simulink model "Satellite_Attitude_Model"  (R2018b)
settings: Solver=ode23tb  StartTime=0.0  StopTime=1000  FixedStep=0.001  RelTol=1e-4
values from neighbouring files (symbols this model uses):
  A = [A11, A12; A21, A22]    [Satellite_Attitude_Model_Parameters.m]
  ArgOfPerigee_init = deg2rad (TLE_degree(5))    [Satellite_Attitude_Model_Parameters.m]
  b = 10e-6    (= 1e-05)    [Satellite_Attitude_Model_Parameters.m]
  B = [B11,B12; B21,B22]    [Satellite_Attitude_Model_Parameters.m]
  D = 0    [Satellite_Attitude_Model_Parameters.m]
  eccentricity_init = TLE_degree(4)    [Satellite_Attitude_Model_Parameters.m]
  Hconf4 = [Hgyro;Hstr]    [Satellite_Attitude_Model_Parameters.m]
  inclination_init = deg2rad (TLE_degree(2))    [Satellite_Attitude_Model_Parameters.m]
  Km = 0.1    [Satellite_Attitude_Model_Parameters.m]
  Kt = 0.1    [Satellite_Attitude_Model_Parameters.m]
  L = 5.2e-3    (= 0.0052)    [Satellite_Attitude_Model_Parameters.m]
  MeanAnomaly_init = deg2rad (TLE_degree(6))    [Satellite_Attitude_Model_Parameters.m]
  meanMotion_init = meanMotion_init*2*pi/86400    [Satellite_Attitude_Model_Parameters.m]
  Q = 1e-10    [Satellite_Attitude_Model_Parameters.m]
  q_init = [0; 0; 0; 1]    [Satellite_Attitude_Model_Parameters.m]
  R = 2    [Satellite_Attitude_Model_Parameters.m]    (also in dynamicFunctions2.m = 7078000)
  RAAN_init = deg2rad (TLE_degree(3))    [Satellite_Attitude_Model_Parameters.m]
  Rconf4 = [diag(ones(3,1))*Rgyro zeros(3,4);         zeros(4,3) diag(ones(1,4))*Rstr]    [Satellite_Attitude_Model_Parameters.m]
  Rgyro = 1e-12    [Satellite_Attitude_Model_Parameters.m]
  Rstr = 1e-12    [Satellite_Attitude_Model_Parameters.m]
  rw_Inertia = 5e-4    (= 0.0005)    [Satellite_Attitude_Model_Parameters.m]
  RW_Mmax = 0.015    [Satellite_Attitude_Model_Parameters.m]
  rw_SensorToBody = [0 0.4741 0.4741 -0.9482;                   -0.9999 0.3333 0.3333 0.3333;                    0 -0.8165 0.8165 0 ]    [Satellite_Attitude_Model_Parameters.m]
  RW_wmax = 300    [Satellite_Attitude_Model_Parameters.m]
  satInertia = [Isx 0 0 ; 0 Isy 0 ; 0 0 Isz]    [Satellite_Attitude_Model_Parameters.m]    (also in dynamicFunctions2.m = diag([Isx Isy Isz]))
  semimajor_init = sqrt(mu_earth^(1/3)/meanMotion_init^(2/3))    [Satellite_Attitude_Model_Parameters.m]
  Ts = 0.01    [Satellite_Attitude_Model_Parameters.m]
  unit7 = ones(7,1)    [Satellite_Attitude_Model_Parameters.m]
  w_dot_init = [0;0;0]    [Satellite_Attitude_Model_Parameters.m]
  w_init = [0; 0; 0]    [Satellite_Attitude_Model_Parameters.m]
  wRW_init = [0;0;0;0]    [Satellite_Attitude_Model_Parameters.m]
undefined symbols (not defined in the file or in its folder): Continuous, Earth, Time, WGS84
libraries: simulink x14, simulink_extras x13, sharedtransform x8, aerolibutil x2, sharedTrackingLibrary x1, ctrlSharedLib x1, aerolibtransform2 x1, aerolibgravity2 x1
(part 1 of 3)
settings Model: SimulationMode=accelerator  Creator=user  LastModifiedBy=user
settings SolverCC: ZeroCrossControl=DisableAll
settings OptimizationCC: BlockReduction=off  DefaultParameterBehavior=Inlined  BufferReuse=off

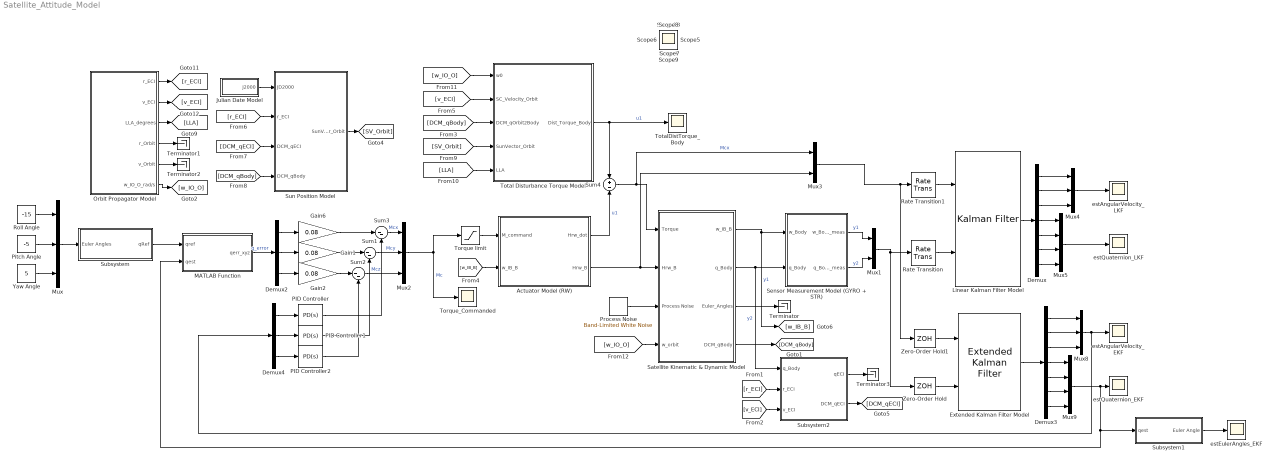
== system Satellite_Attitude_Model ==
  Actuator Model (RW) : Subsystem
  Demux : Demux  Outputs=7
  Demux2 : Demux  Outputs=3
  Demux3 : Demux  Outputs=7
  Demux4 : Demux  Outputs=3
  "Extended Kalman Filter Model " : sharedTrackingLibrary/Extended Kalman Filter  StateTransitionFcn=dynamicFunctions2  HasStateTransitionJacobianFcn=off  HasAdditiveProcessNoise=Additive  ProcessNoise=diag(unit7)*Q  HasTimeVaryingProcessNoise=off  HasStateTransitionFcnExtraArgument=1  InitialState=[w_init; q_init]  InitialStateCovariance=1e-6  MeasurementFcn1=measurementFunction2  HasMeasurementJacobianFcn1=off  HasMeasurementEnablePort1=off  HasAdditiveMeasurementNoise1=Additive  MeasurementNoise1=Rconf4  HasTimeVaryingMeasurementNoise1=off  HasMeasurementFcnExtraArgument1=0  MeasurementFcn2=myMeasurementFcn  HasMeasurementJacobianFcn2=off  HasMeasurementEnablePort2=off  HasAdditiveMeasurementNoise2=Additive  MeasurementNoise2=1  HasTimeVaryingMeasurementNoise2=off  HasMeasurementFcnExtraArgument2=0  MeasurementFcn3=myMeasurementFcn  HasMeasurementJacobianFcn3=off  HasMeasurementEnablePort3=off  HasAdditiveMeasurementNoise3=Additive  MeasurementNoise3=1  HasTimeVaryingMeasurementNoise3=off  HasMeasurementFcnExtraArgument3=0  MeasurementFcn4=myMeasurementFcn  HasMeasurementJacobianFcn4=off  HasMeasurementEnablePort4=off  HasAdditiveMeasurementNoise4=Additive  MeasurementNoise4=1  HasTimeVaryingMeasurementNoise4=off  HasMeasurementFcnExtraArgument4=0  MeasurementFcn5=myMeasurementFcn  HasMeasurementJacobianFcn5=off  HasMeasurementEnablePort5=off  HasAdditiveMeasurementNoise5=Additive  MeasurementNoise5=1  HasTimeVaryingMeasurementNoise5=off  HasMeasurementFcnExtraArgument5=0  EnableMultirate=off  StateTransitionFcnSampleTime=1  MeasurementFcn1SampleTime=1  MeasurementFcn2SampleTime=1  MeasurementFcn3SampleTime=1  MeasurementFcn4SampleTime=1  MeasurementFcn5SampleTime=1  UseCurrentEstimator=on  OutputStateCovariance=off  DataType=double  SampleTime=Ts  NumberOfMeasurements=1
      settings: SourceProductName=Control System Toolbox  SourceProductBaseCode=CT
  Gain1 : Gain  Gain=0.08
  Gain2 : Gain  Gain=0.08
  Gain6 : Gain  Gain=0.08
  Julian Date Model : Subsystem
  Linear Kalman Filter Model : ctrlSharedLib/Kalman Filter  TimeDomain=Continuous-Time  UseCurrentEstimator=on  ModelSource=Individual A, B, C, D matrices  ModelSourceVariable=ss(0.95,1,1,0,1)  A=A  B=B  C=Hconf4  D=D  NumberOfStates=1  NumberOfInputs=1  NumberOfOutputs=1  InitialEstimateSource=Dialog  X0=[w_init; q_init]  P0=10  UseK=off  UseGH=off  NumberOfProcessNoiseInputs=1  G=1  TimeInvariantG=on  H=0  TimeInvariantH=on  Q=diag(unit7)*Q  TimeInvariantQ=on  R=Rconf4  TimeInvariantR=on  N=0  TimeInvariantN=on  AddInputPort=on  AddEnablePort=off  OutputEstimatedY=off  OutputP=off  Ts=-1
      settings: SourceProductBaseCode=CT
  MATLAB Function : MATLAB Function  TreatAsAtomicUnit=on
  Mux{,2,4,8} (4 alike) : Mux  Inputs=3
  Mux1 : Mux  Inputs=2
  Mux3 : Mux  Inputs=2
  Mux5 : Mux
  Mux9 : Mux
  Orbit Propagator Model : Subsystem
  PID Controller : simulink/Continuous/PID Controller  Controller=PD  Form=Parallel  TimeDomain=Continuous-time  SampleTime=-1  IntegratorMethod=Forward Euler  FilterMethod=Forward Euler  ControllerParametersSource=internal  P=1  I=2  D=2  UseFilter=on  N=100  TunerSelectOption=Transfer Function Based (PID Tuner App)  InitialConditionSource=internal  InitialConditionForIntegrator=0  InitialConditionForFilter=0  DifferentiatorICPrevScaledInput=0  ExternalReset=none  TrackingMode=off  Kt=1  LimitOutput=off  UpperSaturationLimit=inf  LowerSaturationLimit=-inf  LinearizeAsGain=on  AntiWindupMode=none  Kb=1  POutMin=[]  POutMax=[]  IOutMin=[]  IOutMax=[]  DOutMin=[]  DOutMax=[]  NOutMin=[]  NOutMax=[]  SumOutMin=[]  SumOutMax=[]  SaturationOutMin=[]  SaturationOutMax=[]  PParamMin=[]  PParamMax=[]  IParamMin=[]  IParamMax=[]  DParamMin=[]  DParamMax=[]  NParamMin=[]  NParamMax=[]  KbParamMin=[]  KbParamMax=[]  KtParamMin=[]  KtParamMax=[]  KbOutMin=[]  KbOutMax=[]  KtOutMin=[]  KtOutMax=[]  IntegratorOutMin=[]  IntegratorOutMax=[]  FilterOutMin=[]  FilterOutMax=[]  SumI1OutMin=[]  SumI1OutMax=[]  SumI2OutMin=[]  SumI2OutMax=[]  SumI3OutMin=[]  SumI3OutMax=[]  SumI4OutMin=[]  SumI4OutMax=[]  SumDOutMin=[]  SumDOutMax=[]  DifferentiatorOutMin=[]  DifferentiatorOutMax=[]  FilterDiffOutCoefMin=[]  FilterDiffOutCoefMax=[]  ReciprocalOutMin=[]  ReciprocalOutMax=[]  SumDenOutMin=[]  SumDenOutMax=[]  SumNumOutMin=[]  SumNumOutMax=[]  DivideOutMin=[]  DivideOutMax=[]  IntegratorContinuousStateAttributes=''  IntegratorStateMustResolveToSignalObject=off  IntegratorRTWStateStorageClass=Auto  FilterContinuousStateAttributes=''  FilterStateMustResolveToSignalObject=off  FilterRTWStateStorageClass=Auto  ParallelPVariant=InternalParameters  IdealPVariant=Disabled  IVariant=Disabled  DVariant=InternalParameters  IntegratorVariant=Disabled  SatVariant=Disabled  AWVariant=Disabled  PCopyVariant=Disabled  TRVariant=Disabled  FdbkBlocksVariant=Forward  IdealPFdbkVariant=Disabled  SatFdbkVariant=Disabled  DerivativeFilterVariant=ContFilter  NVariant=InternalParameters  NCopyVariant=Disabled  FilterICVariant=InternalICsFilter  IntegratorICVariant=Disabled  ExternalResetVariant=Disabled  TRSumVariant=Passthrough  SumFdbkVariant=Disabled  SumVariant=Sum_PD
  PID Controller1 : simulink/Continuous/PID Controller  Controller=PD  Form=Parallel  TimeDomain=Continuous-time  SampleTime=-1  IntegratorMethod=Forward Euler  FilterMethod=Forward Euler  ControllerParametersSource=internal  P=1  I=2  D=2  UseFilter=on  N=100  TunerSelectOption=Transfer Function Based (PID Tuner App)  InitialConditionSource=internal  InitialConditionForIntegrator=0  InitialConditionForFilter=0  DifferentiatorICPrevScaledInput=0  ExternalReset=none  TrackingMode=off  Kt=1  LimitOutput=off  UpperSaturationLimit=inf  LowerSaturationLimit=-inf  LinearizeAsGain=on  AntiWindupMode=none  Kb=1  POutMin=[]  POutMax=[]  IOutMin=[]  IOutMax=[]  DOutMin=[]  DOutMax=[]  NOutMin=[]  NOutMax=[]  SumOutMin=[]  SumOutMax=[]  SaturationOutMin=[]  SaturationOutMax=[]  PParamMin=[]  PParamMax=[]  IParamMin=[]  IParamMax=[]  DParamMin=[]  DParamMax=[]  NParamMin=[]  NParamMax=[]  KbParamMin=[]  KbParamMax=[]  KtParamMin=[]  KtParamMax=[]  KbOutMin=[]  KbOutMax=[]  KtOutMin=[]  KtOutMax=[]  IntegratorOutMin=[]  IntegratorOutMax=[]  FilterOutMin=[]  FilterOutMax=[]  SumI1OutMin=[]  SumI1OutMax=[]  SumI2OutMin=[]  SumI2OutMax=[]  SumI3OutMin=[]  SumI3OutMax=[]  SumI4OutMin=[]  SumI4OutMax=[]  SumDOutMin=[]  SumDOutMax=[]  DifferentiatorOutMin=[]  DifferentiatorOutMax=[]  FilterDiffOutCoefMin=[]  FilterDiffOutCoefMax=[]  ReciprocalOutMin=[]  ReciprocalOutMax=[]  SumDenOutMin=[]  SumDenOutMax=[]  SumNumOutMin=[]  SumNumOutMax=[]  DivideOutMin=[]  DivideOutMax=[]  IntegratorContinuousStateAttributes=''  IntegratorStateMustResolveToSignalObject=off  IntegratorRTWStateStorageClass=Auto  FilterContinuousStateAttributes=''  FilterStateMustResolveToSignalObject=off  FilterRTWStateStorageClass=Auto  ParallelPVariant=InternalParameters  IdealPVariant=Disabled  IVariant=Disabled  DVariant=InternalParameters  IntegratorVariant=Disabled  SatVariant=Disabled  AWVariant=Disabled  PCopyVariant=Disabled  TRVariant=Disabled  FdbkBlocksVariant=Forward  IdealPFdbkVariant=Disabled  SatFdbkVariant=Disabled  DerivativeFilterVariant=ContFilter  NVariant=InternalParameters  NCopyVariant=Disabled  FilterICVariant=InternalICsFilter  IntegratorICVariant=Disabled  ExternalResetVariant=Disabled  TRSumVariant=Passthrough  SumFdbkVariant=Disabled  SumVariant=Sum_PD
  PID Controller2 : simulink/Continuous/PID Controller  Controller=PD  Form=Parallel  TimeDomain=Continuous-time  SampleTime=-1  IntegratorMethod=Forward Euler  FilterMethod=Forward Euler  ControllerParametersSource=internal  P=1  I=2  D=2  UseFilter=on  N=100  TunerSelectOption=Transfer Function Based (PID Tuner App)  InitialConditionSource=internal  InitialConditionForIntegrator=0  InitialConditionForFilter=0  DifferentiatorICPrevScaledInput=0  ExternalReset=none  TrackingMode=off  Kt=1  LimitOutput=off  UpperSaturationLimit=inf  LowerSaturationLimit=-inf  LinearizeAsGain=on  AntiWindupMode=none  Kb=1  POutMin=[]  POutMax=[]  IOutMin=[]  IOutMax=[]  DOutMin=[]  DOutMax=[]  NOutMin=[]  NOutMax=[]  SumOutMin=[]  SumOutMax=[]  SaturationOutMin=[]  SaturationOutMax=[]  PParamMin=[]  PParamMax=[]  IParamMin=[]  IParamMax=[]  DParamMin=[]  DParamMax=[]  NParamMin=[]  NParamMax=[]  KbParamMin=[]  KbParamMax=[]  KtParamMin=[]  KtParamMax=[]  KbOutMin=[]  KbOutMax=[]  KtOutMin=[]  KtOutMax=[]  IntegratorOutMin=[]  IntegratorOutMax=[]  FilterOutMin=[]  FilterOutMax=[]  SumI1OutMin=[]  SumI1OutMax=[]  SumI2OutMin=[]  SumI2OutMax=[]  SumI3OutMin=[]  SumI3OutMax=[]  SumI4OutMin=[]  SumI4OutMax=[]  SumDOutMin=[]  SumDOutMax=[]  DifferentiatorOutMin=[]  DifferentiatorOutMax=[]  FilterDiffOutCoefMin=[]  FilterDiffOutCoefMax=[]  ReciprocalOutMin=[]  ReciprocalOutMax=[]  SumDenOutMin=[]  SumDenOutMax=[]  SumNumOutMin=[]  SumNumOutMax=[]  DivideOutMin=[]  DivideOutMax=[]  IntegratorContinuousStateAttributes=''  IntegratorStateMustResolveToSignalObject=off  IntegratorRTWStateStorageClass=Auto  FilterContinuousStateAttributes=''  FilterStateMustResolveToSignalObject=off  FilterRTWStateStorageClass=Auto  ParallelPVariant=InternalParameters  IdealPVariant=Disabled  IVariant=Disabled  DVariant=InternalParameters  IntegratorVariant=Disabled  SatVariant=Disabled  AWVariant=Disabled  PCopyVariant=Disabled  TRVariant=Disabled  FdbkBlocksVariant=Forward  IdealPFdbkVariant=Disabled  SatFdbkVariant=Disabled  DerivativeFilterVariant=ContFilter  NVariant=InternalParameters  NCopyVariant=Disabled  FilterICVariant=InternalICsFilter  IntegratorICVariant=Disabled  ExternalResetVariant=Disabled  TRSumVariant=Passthrough  SumFdbkVariant=Disabled  SumVariant=Sum_PD
  Pitch Angle : Constant  Value=-5
  Process Noise : simulink/Sources/Band-Limited White Noise  Cov=Q*Ts  Ts=Ts  seed=[23341]
  Rate Transition : RateTransition  OutPortSampleTimeOpt=Inherit  OutPortSampleTime=Ts
  Rate Transition1 : RateTransition  OutPortSampleTimeOpt=Inherit  OutPortSampleTime=Ts
  Roll Angle : Constant  Value=-15
  Satellite Kinematic & Dynamic Model : Subsystem
  Sensor Measurement Model (GYRO + STR) : Subsystem
  Subsystem : Subsystem
  Subsystem1 : Subsystem
  Subsystem2 : Subsystem
  Sum1 : Sum  Inputs=|--
  Sum2 : Sum  Inputs=|--
  Sum3 : Sum  Inputs=|--
  Sum4 : Sum  Inputs=+|-
  Sun Position Model : Subsystem
  Terminator{,1..3} (4 alike) : Terminator
  Torque limit : Saturate  UpperLimit=RW_Mmax  LowerLimit=-RW_Mmax
  Torque_Commanded : Scope
  Total Disturbance Torque Model : Subsystem
  TotalDistTorque_Body : Scope
  Yaw Angle : Constant  Value=5
  Zero-Order Hold : ZeroOrderHold  SampleTime=Ts
  Zero-Order Hold1 : ZeroOrderHold  SampleTime=Ts
  estAngularVelocity_EKF : Scope
  estAngularVelocity_LKF : Scope
  estEulerAngles_EKF : Scope
  "estQuaternion_EKF " : Scope
  estQuaternion_LKF : Scope
  Scope{1,3,5..9,13} (8 alike) : Scope
  wires:
  Linear Kalman Filter Model/1 -> Demux/1
  Demux/1 -> Mux4/1
  Demux/2 -> Mux4/2
  Demux/3 -> Mux4/3
  Mux4/1 -> estAngularVelocity_LKF/1
  Demux/4 -> Mux5/1
  Demux/5 -> Mux5/2
  Demux/6 -> Mux5/3
  Demux/7 -> Mux5/4
  Mux5/1 -> estQuaternion_LKF/1
  Demux3/1 -> Mux8/1
  Demux3/2 -> Mux8/2
  Demux3/3 -> Mux8/3
  Demux3/4 -> Mux9/1
  Demux3/5 -> Mux9/2
  Demux3/7 -> Mux9/4
  Demux3/6 -> Mux9/3
  Zero-Order Hold/1 -> "Extended Kalman Filter Model "/2
  Zero-Order Hold1/1 -> "Extended Kalman Filter Model "/1
  Total Disturbance Torque Model/1(Dist_Torque_Body) -> TotalDistTorque_Body/1, Sum4/1  "u1"
  [w_IO_O] -> Satellite Kinematic & Dynamic Model/4(w_orbit)
  Satellite Kinematic & Dynamic Model/4(DCM_qBody) -> [DCM_qBody]
  Sun Position Model/1(SunVector_Orbit) -> [SV_Orbit]
  [v_ECI] -> Total Disturbance Torque Model/2(SC_Velocity_Orbit)
  [SV_Orbit] -> Total Disturbance Torque Model/4(SunVector_Orbit)
  Julian Date Model/1(J2000) -> Sun Position Model/1(JD2000)
  [r_ECI] -> Sun Position Model/2(r_ECI)
  [DCM_qBody] -> Total Disturbance Torque Model/3(DCM_qOrbit2Body)
  Satellite Kinematic & Dynamic Model/3(Euler_Angles) -> Terminator/1
  Subsystem2/1(qECI) -> Terminator3/1
  [r_ECI] -> Subsystem2/2(r_ECI)
  [v_ECI] -> Subsystem2/3(v_ECI)
  Mux1/1 -> Rate Transition/1, Zero-Order Hold/1
  Rate Transition/1 -> Linear Kalman Filter Model/2
  Rate Transition1/1 -> Linear Kalman Filter Model/1
  "Extended Kalman Filter Model "/1 -> Demux3/1
  [w_IB_B] -> Actuator Model (RW)/2(w_IB_B)
  Mux2/1 -> Torque limit/1, Torque_Commanded/1  "Mc"
  Mux9/1 -> "estQuaternion_EKF "/1, Subsystem1/1(qest), MATLAB Function/2(qest)
  Mux8/1 -> Demux4/1, estAngularVelocity_EKF/1
  Process Noise/1 -> Satellite Kinematic & Dynamic Model/3("Process Noise ")
  Satellite Kinematic & Dynamic Model/1(w_IB_B) -> Sensor Measurement Model (GYRO + STR)/1(w_Body), [w_IB_B]  "y1"
  Satellite Kinematic & Dynamic Model/2(q_Body) -> Sensor Measurement Model (GYRO + STR)/2(q_Body), Subsystem2/1("q_Body ")  "y2"
  Sensor Measurement Model (GYRO + STR)/1(w_Body_meas) -> Mux1/1  "y1"
  Sensor Measurement Model (GYRO + STR)/2(q_Body_meas) -> Mux1/2  "y2"
  Actuator Model (RW)/1("Hrw_dot ") -> Sum4/2  "u1"
  Torque limit/1 -> Actuator Model (RW)/1("M_command ")
  Roll Angle/1 -> Mux/1
  Yaw Angle/1 -> Mux/3
  Pitch Angle/1 -> Mux/2
  Mux/1 -> Subsystem/1(Euler Angles)
  Subsystem/1(qRef) -> MATLAB Function/1(qref)
  Subsystem1/1(Euler Angle) -> estEulerAngles_EKF/1
  Orbit Propagator Model/3("LLA_degrees ") -> [LLA]
  Orbit Propagator Model/2("v_ECI ") -> [v_ECI]
  Orbit Propagator Model/1(r_ECI) -> [r_ECI]
  Subsystem2/2(DCM_qECI) -> [DCM_qECI]
  [DCM_qECI] -> Sun Position Model/3(DCM_qECI)
  [DCM_qBody] -> Sun Position Model/4(DCM_qBody)
  [LLA] -> Total Disturbance Torque Model/5(LLA)
  Orbit Propagator Model/4(r_Orbit) -> Terminator1/1
  Orbit Propagator Model/5(v_Orbit) -> Terminator2/1
  MATLAB Function/1(qerr_xyz) -> Demux2/1  "q_error"
  Demux2/1 -> Gain6/1
  Demux2/2 -> Gain1/1
  Demux2/3 -> Gain2/1
  Gain6/1 -> Sum3/1
  Gain1/1 -> Sum1/1
  Gain2/1 -> Sum2/1
  Demux4/3 -> PID Controller2/1
  Demux4/2 -> PID Controller1/1
  PID Controller1/1 -> Sum1/2
  Demux4/1 -> PID Controller/1
  PID Controller/1 -> Sum3/2
  PID Controller2/1 -> Sum2/2
  Sum3/1 -> Mux2/1  "Mcx"
  Sum1/1 -> Mux2/2  "Mcy"
  Sum2/1 -> Mux2/3  "Mcz"
  Sum4/1 -> Mux3/1, Satellite Kinematic & Dynamic Model/1(Torque)  "Mcx"
  Orbit Propagator Model/6(w_IO_O_rad/s) -> [w_IO_O]
  [w_IO_O] -> Total Disturbance Torque Model/1("w0 ")
  Actuator Model (RW)/2(Hrw_B) -> Satellite Kinematic & Dynamic Model/2(Hrw_B), Mux3/2
  Mux3/1 -> Zero-Order Hold1/1, Rate Transition1/1

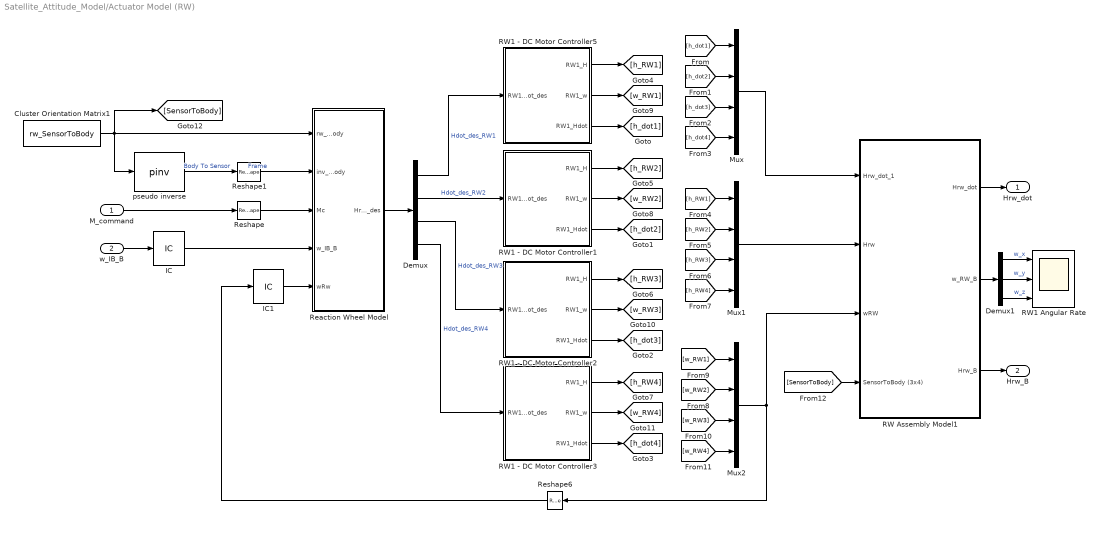
== system Satellite_Attitude_Model/Actuator Model (RW) ==
  "M_command " : Inport
  w_IB_B : Inport  Port=2
  Cluster Orientation Matrix1 : Constant  Value=rw_SensorToBody  VectorParams1D=off  SampleTime=Ts
  Demux : Demux
  Demux1 : Demux  Outputs=3
  IC : InitialCondition  Value=w_init
  IC1 : InitialCondition  Value=wRW_init
  Mux : Mux
  Mux1 : Mux
  Mux2 : Mux
  RW Assembly Model1 : Subsystem
  RW1 - DC Motor Controller1 : Subsystem
  RW1 - DC Motor Controller2 : Subsystem
  RW1 - DC Motor Controller3 : Subsystem
  RW1 - DC Motor Controller5 : Subsystem
  RW1 Angular Rate : Scope  NumInputPorts=3
  Reaction Wheel Model : MATLAB Function  TreatAsAtomicUnit=on
  Reshape : Reshape  OutputDimensionality=Column vector (2-D)
  Reshape1 : Reshape  OutputDimensionality=Customize  OutputDimensions=[4,3]
  Reshape6 : Reshape  OutputDimensionality=Column vector (2-D)
  pseudo inverse : MATLABFcn  MATLABFcn=pinv
  "Hrw_dot " : Outport
  Hrw_B : Outport  Port=2
  wires:
  Demux/1 -> RW1 - DC Motor Controller5/1(RW1_Hdot_des)  "Hdot_des_RW1"
  Demux/2 -> RW1 - DC Motor Controller1/1(RW1_Hdot_des)  "Hdot_des_RW2"
  Demux/3 -> RW1 - DC Motor Controller2/1(RW1_Hdot_des)  "Hdot_des_RW3"
  Demux/4 -> RW1 - DC Motor Controller3/1(RW1_Hdot_des)  "Hdot_des_RW4"
  Demux1/3 -> RW1 Angular Rate/3  "w_z"
  Demux1/1 -> RW1 Angular Rate/1  "w_x"
  Demux1/2 -> RW1 Angular Rate/2  "w_y"
  "M_command "/1 -> Reshape/1
  Reaction Wheel Model/1(Hrw_dot_des) -> Demux/1
  [h_dot1] -> Mux/1
  [h_dot2] -> Mux/2
  [h_dot3] -> Mux/3
  [h_dot4] -> Mux/4
  Mux/1 -> RW Assembly Model1/1(Hrw_dot_1)
  [h_RW1] -> Mux1/1
  [h_RW2] -> Mux1/2
  [h_RW3] -> Mux1/3
  [h_RW4] -> Mux1/4
  Mux1/1 -> RW Assembly Model1/2(Hrw)
  [w_RW2] -> Mux2/2
  [w_RW1] -> Mux2/1
  [w_RW3] -> Mux2/3
  [w_RW4] -> Mux2/4
  pseudo inverse/1 -> Reshape1/1  "Body To Sensor         Frame"
  Reshape/1 -> Reaction Wheel Model/3(Mc)
  Cluster Orientation Matrix1/1 -> pseudo inverse/1, [SensorToBody], Reaction Wheel Model/1(rw_SensorToBody)
  [SensorToBody] -> RW Assembly Model1/4(SensorToBody (3x4))
  RW Assembly Model1/2(w_RW_B) -> Demux1/1
  RW Assembly Model1/1(Hrw_dot) -> "Hrw_dot "/1
  Mux2/1 -> Reshape6/1, RW Assembly Model1/3(wRW)
  Reshape6/1 -> IC1/1
  Reshape1/1 -> Reaction Wheel Model/2(inv_rwSensorToBody)
  w_IB_B/1 -> IC/1
  IC/1 -> Reaction Wheel Model/4(w_IB_B)
  IC1/1 -> Reaction Wheel Model/5(wRw)
  RW1 - DC Motor Controller5/2(RW1_w) -> [w_RW1]
  RW1 - DC Motor Controller5/1(RW1_H) -> [h_RW1]
  RW1 - DC Motor Controller5/3(RW1_Hdot) -> [h_dot1]
  RW1 - DC Motor Controller1/1(RW1_H) -> [h_RW2]
  RW1 - DC Motor Controller1/2(RW1_w) -> [w_RW2]
  RW1 - DC Motor Controller1/3(RW1_Hdot) -> [h_dot2]
  RW1 - DC Motor Controller2/1(RW1_H) -> [h_RW3]
  RW1 - DC Motor Controller2/2(RW1_w) -> [w_RW3]
  RW1 - DC Motor Controller2/3(RW1_Hdot) -> [h_dot3]
  RW1 - DC Motor Controller3/1(RW1_H) -> [h_RW4]
  RW1 - DC Motor Controller3/2(RW1_w) -> [w_RW4]
  RW1 - DC Motor Controller3/3(RW1_Hdot) -> [h_dot4]
  RW Assembly Model1/3(Hrw_B) -> Hrw_B/1

== system Satellite_Attitude_Model/Julian Date Model ==
  Clk : Clock
  Display : Display
  Display2 : Display
  Epoch1 : Constant  Value=[ 2012 7 22 16 30 24.87]  VectorParams1D=off
  Gain1 : Gain  Gain=1/86400
  Sum2 : Sum  Inputs=|++
  Time To Julian Date Model : Subsystem
  J2000 : Outport
  wires:
  Sum2/1 -> Display2/1, J2000/1
  Gain1/1 -> Sum2/1
  Epoch1/1 -> Time To Julian Date Model/1(time)
  Clk/1 -> Gain1/1
  Time To Julian Date Model/1(JulianDate) -> Sum2/2, Display/1

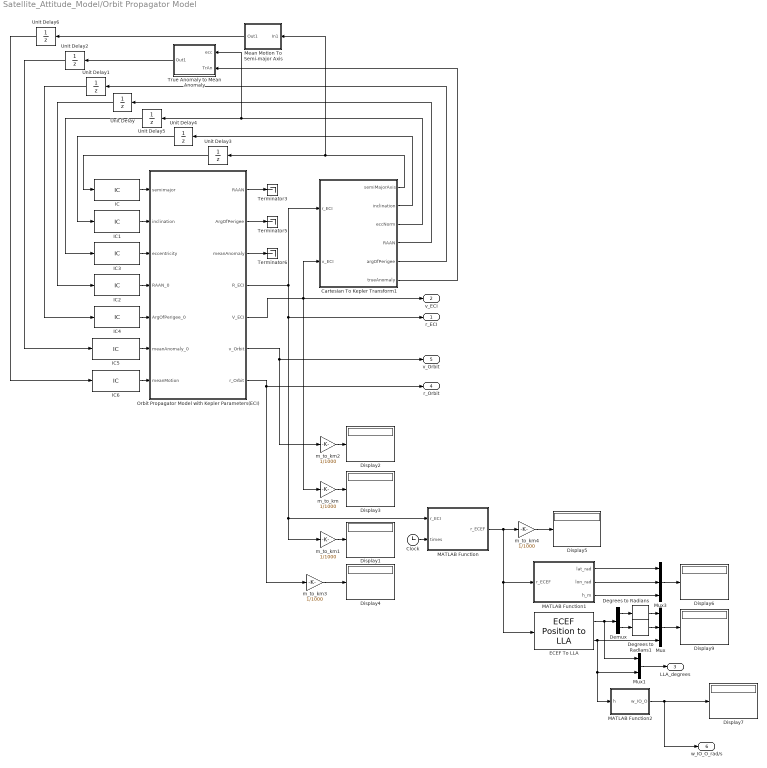
== system Satellite_Attitude_Model/Orbit Propagator Model ==
  Cartesian To Kepler Transform1 : MATLAB Function  TreatAsAtomicUnit=on
  Clock : Clock
  Degrees to Radians : simulink_extras/Transformations/Degrees to Radians
  Degrees to Radians1 : simulink_extras/Transformations/Degrees to Radians
  Demux : Demux  Outputs=2
  Display{1..7,9} (8 alike) : Display
  "ECEF To LLA " : aerolibtransform2/ECEF Position to LLA  units=Metric (MKS)  ptype=Earth (WGS84)  F=1/298.257223563  R=6378137
      settings: SourceProductName=Aerospace Blockset  SourceProductBaseCode=AE
  IC : InitialCondition  Value=semimajor_init
  IC1 : InitialCondition  Value=inclination_init
  IC2 : InitialCondition  Value=RAAN_init
  IC3 : InitialCondition  Value=eccentricity_init
  IC4 : InitialCondition  Value=ArgOfPerigee_init
  IC5 : InitialCondition  Value=MeanAnomaly_init
  IC6 : InitialCondition  Value=meanMotion_init
  MATLAB Function : MATLAB Function  TreatAsAtomicUnit=on
  MATLAB Function1 : MATLAB Function  TreatAsAtomicUnit=on
  MATLAB Function2 : MATLAB Function  TreatAsAtomicUnit=on
  Mean Motion To Semi-major Axis : Subsystem
  Mux : Mux  Inputs=3
  Mux1 : Mux  Inputs=2
  Mux3 : Mux  Inputs=3
  Orbit Propagator Model with Kepler Parameters(ECI) : Subsystem
  Terminator3 : Terminator
  Terminator5 : Terminator
  Terminator6 : Terminator
  True Anomaly to Mean Anomaly : Subsystem
  Unit Delay{,1..6} (7 alike) : UnitDelay  SampleTime=-1
  m_to_km{,1..4} (5 alike) : Gain  Gain=1/1000
  r_ECI : Outport
  "v_ECI " : Outport  Port=2
  "LLA_degrees " : Outport  Port=3
  r_Orbit : Outport  Port=4
  v_Orbit : Outport  Port=5
  w_IO_O_rad/s : Outport  Port=6
  wires:
  IC4/1 -> Orbit Propagator Model with Kepler Parameters(ECI)/5(ArgOfPerigee_0)
  IC2/1 -> Orbit Propagator Model with Kepler Parameters(ECI)/4(RAAN_0)
  IC1/1 -> Orbit Propagator Model with Kepler Parameters(ECI)/2(inclination)
  IC/1 -> Orbit Propagator Model with Kepler Parameters(ECI)/1(semimajor)
  IC3/1 -> Orbit Propagator Model with Kepler Parameters(ECI)/3(eccentricity)
  IC5/1 -> Orbit Propagator Model with Kepler Parameters(ECI)/6(meanAnomaly_0)
  Cartesian To Kepler Transform1/3(eccNorm) -> True Anomaly to Mean Anomaly/1(ecc), Unit Delay5/1
  Cartesian To Kepler Transform1/2(inclination) -> Unit Delay4/1
  Cartesian To Kepler Transform1/4(RAAN) -> Unit Delay/1
  Cartesian To Kepler Transform1/1(semiMajorAxis) -> Mean Motion To Semi-major Axis/1(In1), Unit Delay3/1
  Cartesian To Kepler Transform1/5(argOfPerigee) -> Unit Delay1/1
  Unit Delay3/1 -> IC/1
  Unit Delay4/1 -> IC1/1
  Unit Delay5/1 -> IC3/1
  Orbit Propagator Model with Kepler Parameters(ECI)/4(R_ECI) -> Cartesian To Kepler Transform1/1(r_ECI), MATLAB Function/1(r_ECI), m_to_km1/1, r_ECI/1
  Orbit Propagator Model with Kepler Parameters(ECI)/5(V_ECI) -> m_to_km/1, "v_ECI "/1, Cartesian To Kepler Transform1/2(v_ECI)
  m_to_km1/1 -> Display1/1
  m_to_km/1 -> Display3/1
  m_to_km2/1 -> Display2/1
  Orbit Propagator Model with Kepler Parameters(ECI)/6(v_Orbit) -> m_to_km2/1, v_Orbit/1
  m_to_km3/1 -> Display4/1
  Clock/1 -> MATLAB Function/2(times)
  MATLAB Function/1(r_ECEF) -> "ECEF To LLA "/1, MATLAB Function1/1(r_ECEF), m_to_km4/1
  m_to_km4/1 -> Display5/1
  Orbit Propagator Model with Kepler Parameters(ECI)/7(r_Orbit) -> r_Orbit/1, m_to_km3/1
  Orbit Propagator Model with Kepler Parameters(ECI)/1(RAAN) -> Terminator3/1
  Orbit Propagator Model with Kepler Parameters(ECI)/3(meanAnomaly) -> Terminator6/1
  Orbit Propagator Model with Kepler Parameters(ECI)/2(ArgOfPerigee) -> Terminator5/1
  Unit Delay/1 -> IC2/1
  Unit Delay1/1 -> IC4/1
  Unit Delay2/1 -> IC5/1
  "ECEF To LLA "/1 -> Mux1/1, Demux/1
  "ECEF To LLA "/2 -> Mux/3, MATLAB Function2/1(h), Mux1/2
  Mux/1 -> Display9/1
  Demux/1 -> Degrees to Radians/1
  Demux/2 -> Degrees to Radians1/1
  Degrees to Radians/1 -> Mux/1
  Degrees to Radians1/1 -> Mux/2
  Mux1/1 -> "LLA_degrees "/1
  MATLAB Function1/1(lat_rad) -> Mux3/1
  MATLAB Function1/2(lon_rad) -> Mux3/2
  Mux3/1 -> Display6/1
  MATLAB Function1/3(h_m) -> Mux3/3
  MATLAB Function2/1(w_IO_O) -> w_IO_O_rad/s/1, Display7/1
  IC6/1 -> Orbit Propagator Model with Kepler Parameters(ECI)/7(meanMotion)
  Mean Motion To Semi-major Axis/1(Out1) -> Unit Delay6/1
  Unit Delay6/1 -> IC6/1
  Cartesian To Kepler Transform1/6(trueAnomaly) -> True Anomaly to Mean Anomaly/2(TrAn)
  True Anomaly to Mean Anomaly/1(Out1) -> Unit Delay2/1

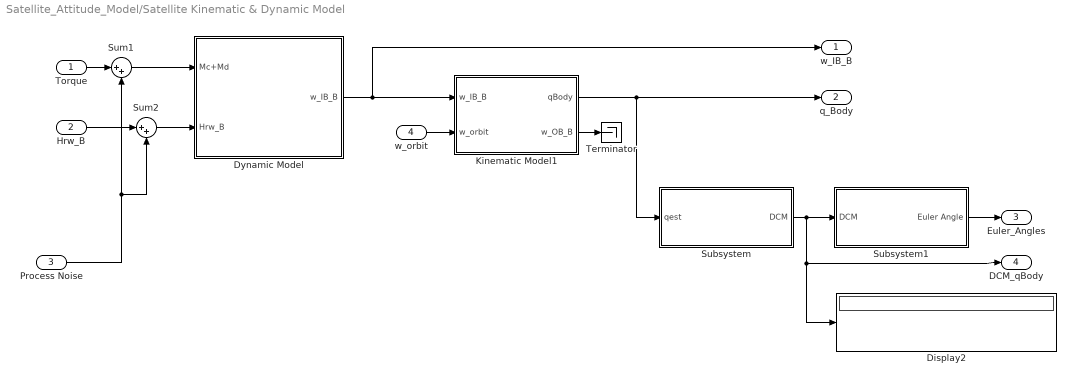
== system Satellite_Attitude_Model/Satellite Kinematic & Dynamic Model ==
  Torque : Inport
  Hrw_B : Inport  Port=2
  "Process Noise " : Inport  Port=3
  w_orbit : Inport  Port=4
  Display2 : Display
  Dynamic Model : Subsystem
  Kinematic Model1 : Subsystem
  Subsystem : Subsystem
  Subsystem1 : Subsystem
  Sum1 : Sum  Inputs=|++
  Sum2 : Sum  Inputs=|++
  Terminator : Terminator
  w_IB_B : Outport
  q_Body : Outport  Port=2
  Euler_Angles : Outport  Port=3
  DCM_qBody : Outport  Port=4
  wires:
  Kinematic Model1/1(qBody) -> Subsystem/1(qest), q_Body/1
  w_orbit/1 -> Kinematic Model1/2(w_orbit)
  "Process Noise "/1 -> Sum2/2, Sum1/2
  Torque/1 -> Sum1/1
  Sum1/1 -> Dynamic Model/1(Mc+Md)
  Kinematic Model1/2(w_OB_B) -> Terminator/1
  Dynamic Model/1(w_IB_B) -> Kinematic Model1/1(w_IB_B), w_IB_B/1
  Subsystem/1("DCM ") -> Display2/1, DCM_qBody/1, Subsystem1/1("DCM ")
  Subsystem1/1(Euler Angle) -> Euler_Angles/1
  Hrw_B/1 -> Sum2/1
  Sum2/1 -> Dynamic Model/2("Hrw_B ")

== system Satellite_Attitude_Model/Sensor Measurement Model (GYRO + STR) ==
  w_Body : Inport
  q_Body : Inport  Port=2
  GYRO Sensor Model : Subsystem
  Normalization Model : Subsystem
  Star Tracker Model : Subsystem
  w_Body_meas : Outport
  q_Body_meas : Outport  Port=2
  wires:
  GYRO Sensor Model/1(w_Body_meas) -> w_Body_meas/1
  w_Body/1 -> GYRO Sensor Model/1(w_Body)
  q_Body/1 -> Star Tracker Model/1(q_Body)
  Normalization Model/1(Normalized_u) -> q_Body_meas/1
  Star Tracker Model/1(q_Body_meas) -> Normalization Model/1(u)

== system Satellite_Attitude_Model/Subsystem ==
  Euler Angles : Inport
  Degrees to Radians1 : simulink_extras/Transformations/Degrees to Radians
  Direction Cosine Matrix to Quaternions : sharedtransform/Direction Cosine Matrix  to Quaternions  aMode=0  action=None  tolerance=eps(2)
      settings: SourceProductName=Aerospace Blockset  SourceProductBaseCode=AE
  Rotation Angles to Direction Cosine Matrix : sharedtransform/Rotation Angles to Direction Cosine Matrix  rotationOrder=ZYX  aMode=aMode
      settings: SourceProductBaseCode=AE
  Subsystem1 : Subsystem
  qRef : Outport
  wires:
  Euler Angles/1 -> Degrees to Radians1/1
  Degrees to Radians1/1 -> Rotation Angles to Direction Cosine Matrix/1
  Rotation Angles to Direction Cosine Matrix/1 -> Direction Cosine Matrix to Quaternions/1
  Direction Cosine Matrix to Quaternions/1 -> Subsystem1/1(q0,q1,q2,q3)
  Subsystem1/1(q1,q2,q3,q4) -> qRef/1

== system Satellite_Attitude_Model/Subsystem1 ==
  qest : Inport
  Demux2 : Demux
  Mux2 : Mux
  Quaternions to Rotation Angles : sharedtransform/Quaternions to Rotation Angles  rotationOrder=ZYX  aMode=aMode
      settings: SourceProductBaseCode=AE
  Radians to Degrees1 : simulink_extras/Transformations/Radians to Degrees
  Euler Angle : Outport
  wires:
  Quaternions to Rotation Angles/1 -> Radians to Degrees1/1
  Radians to Degrees1/1 -> Euler Angle/1
  Demux2/3 -> Mux2/4
  Mux2/1 -> Quaternions to Rotation Angles/1
  qest/1 -> Demux2/1
  Demux2/4 -> Mux2/1
  Demux2/2 -> Mux2/3
  Demux2/1 -> Mux2/2

== system Satellite_Attitude_Model/Subsystem2 ==
  "q_Body " : Inport
  r_ECI : Inport  Port=2
  v_ECI : Inport  Port=3
  Demux : Demux
  Direction Cosine Matrix to Quaternions : sharedtransform/Direction Cosine Matrix  to Quaternions  aMode=0  action=None  tolerance=eps(2)
      settings: SourceProductName=Aerospace Blockset  SourceProductBaseCode=AE
  MATLAB Function : MATLAB Function  TreatAsAtomicUnit=on
  MATLAB Function2 : MATLAB Function  TreatAsAtomicUnit=on
  Mux : Mux
  Subsystem : Subsystem
  qECI : Outport
  DCM_qECI : Outport  Port=2
  wires:
  MATLAB Function2/1(q_DCM) -> Direction Cosine Matrix to Quaternions/1
  Direction Cosine Matrix to Quaternions/1 -> Demux/1
  Demux/3 -> Mux/2
  "q_Body "/1 -> MATLAB Function/2(p)
  Demux/1 -> Mux/4
  Demux/2 -> Mux/1
  Demux/4 -> Mux/3
  MATLAB Function/1(y) -> Subsystem/1(qest), qECI/1
  Mux/1 -> MATLAB Function/1(q)
  r_ECI/1 -> MATLAB Function2/1(r_ECI)
  v_ECI/1 -> MATLAB Function2/2(v_ECI)
  Subsystem/1("DCM ") -> DCM_qECI/1

== system Satellite_Attitude_Model/Sun Position Model ==
  JD2000 : Inport
  r_ECI : Inport  Port=2
  DCM_qECI : Inport  Port=3
  DCM_qBody : Inport  Port=4
  Subsystem1 : Subsystem
  Terminator1 : Terminator
  SunVector_Orbit : Outport
  wires:
  JD2000/1 -> Subsystem1/1(JD2000)
  r_ECI/1 -> Subsystem1/2(r_ECI)
  DCM_qECI/1 -> Subsystem1/3(DCM_qECI)
  DCM_qBody/1 -> Subsystem1/4(DCM_qBody)
  Subsystem1/1(SunVector_Orbit) -> SunVector_Orbit/1
  Subsystem1/2("sunVector_ECI ") -> Terminator1/1

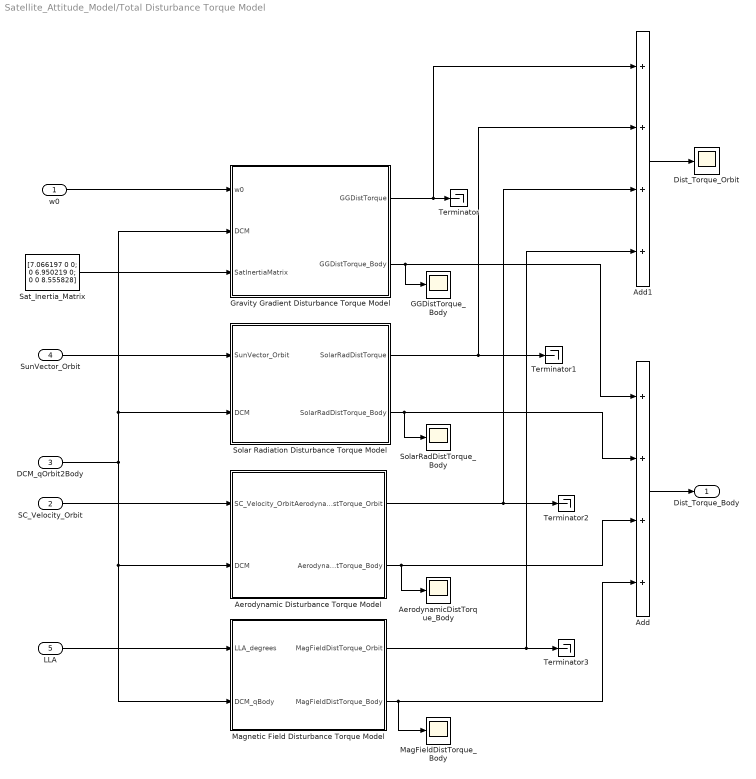
== system Satellite_Attitude_Model/Total Disturbance Torque Model ==
  "w0 " : Inport
  SC_Velocity_Orbit : Inport  Port=2
  DCM_qOrbit2Body : Inport  Port=3
  SunVector_Orbit : Inport  Port=4
  LLA : Inport  Port=5
  Add : Sum  Inputs=++++
  Add1 : Sum  Inputs=++++
  Aerodynamic Disturbance Torque Model : Subsystem
  AerodynamicDistTorque_Body : Scope
  Dist_Torque_Orbit : Scope
  GGDistTorque_Body : Scope
  Gravity Gradient Disturbance Torque Model : Subsystem
  MagFieldDistTorque_Body : Scope
  Magnetic Field Disturbance Torque Model : Subsystem
  Sat_Inertia_Matrix : Constant  Value=[7.066197 0 0; 0 6.950219 0; 0 0 8.555828]
  Solar Radiation Disturbance Torque Model : Subsystem
  SolarRadDistTorque_Body : Scope
  Terminator{,1..3} (4 alike) : Terminator
  Dist_Torque_Body : Outport
  wires:
  Aerodynamic Disturbance Torque Model/2(AerodynamicDistTorque_Body) -> Add/3, AerodynamicDistTorque_Body/1
  Aerodynamic Disturbance Torque Model/1(AerodynamicDistTorque_Orbit) -> Terminator2/1, Add1/3
  SC_Velocity_Orbit/1 -> Aerodynamic Disturbance Torque Model/1(SC_Velocity_Orbit)
  Solar Radiation Disturbance Torque Model/2(SolarRadDistTorque_Body) -> SolarRadDistTorque_Body/1, Add/2
  Magnetic Field Disturbance Torque Model/1(MagFieldDistTorque_Orbit) -> Terminator3/1, Add1/4
  Gravity Gradient Disturbance Torque Model/1(GGDistTorque) -> Add1/1, Terminator/1
  DCM_qOrbit2Body/1 -> Gravity Gradient Disturbance Torque Model/2(DCM), Solar Radiation Disturbance Torque Model/2(DCM), Magnetic Field Disturbance Torque Model/2(DCM_qBody), Aerodynamic Disturbance Torque Model/2(DCM)
  Magnetic Field Disturbance Torque Model/2(MagFieldDistTorque_Body) -> Add/4, MagFieldDistTorque_Body/1
  "w0 "/1 -> Gravity Gradient Disturbance Torque Model/1(w0)
  Gravity Gradient Disturbance Torque Model/2(GGDistTorque_Body) -> GGDistTorque_Body/1, Add/1
  Add/1 -> Dist_Torque_Body/1
  Sat_Inertia_Matrix/1 -> Gravity Gradient Disturbance Torque Model/3(SatInertiaMatrix)
  SunVector_Orbit/1 -> Solar Radiation Disturbance Torque Model/1(SunVector_Orbit)
  LLA/1 -> Magnetic Field Disturbance Torque Model/1(LLA_degrees)
  Solar Radiation Disturbance Torque Model/1(SolarRadDistTorque) -> Terminator1/1, Add1/2
  Add1/1 -> Dist_Torque_Orbit/1

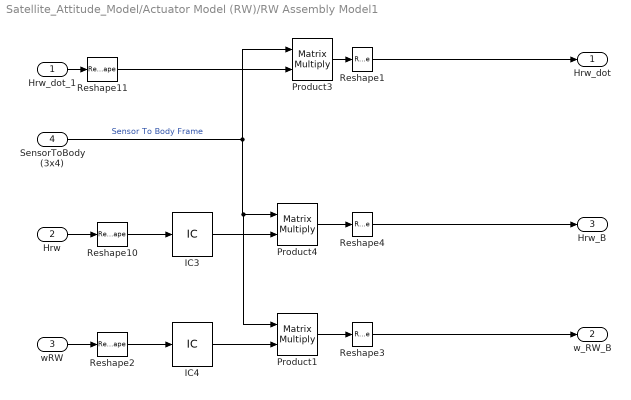
== system Satellite_Attitude_Model/Actuator Model (RW)/RW Assembly Model1 ==
  Hrw_dot_1 : Inport
  Hrw : Inport  Port=2
  wRW : Inport  Port=3
  SensorToBody (3x4) : Inport  Port=4
  IC3 : InitialCondition  Value=[wRW_init(1,1)*rw_Inertia; wRW_init(2,1)*rw_Inertia; wRW_init(3,1)*rw_Inertia;wRW_init(4,1)*rw_Inertia]
  IC4 : InitialCondition  Value=wRW_init
  Product1 : Product  Inputs=**  Multiplication=Matrix(*)  RndMeth=Zero
  Product3 : Product  Inputs=**  Multiplication=Matrix(*)  RndMeth=Zero
  Product4 : Product  Inputs=**  Multiplication=Matrix(*)  RndMeth=Zero
  Reshape{1..4,10..11} (6 alike) : Reshape  OutputDimensionality=Column vector (2-D)
  Hrw_dot : Outport
  w_RW_B : Outport  Port=2
  Hrw_B : Outport  Port=3
  wires:
  SensorToBody (3x4)/1 -> Product3/1, Product1/1, Product4/1  "Sensor To Body Frame"
  Product4/1 -> Reshape4/1
  Reshape1/1 -> Hrw_dot/1
  Reshape4/1 -> Hrw_B/1
  IC3/1 -> Product4/2
  IC4/1 -> Product1/2
  Product1/1 -> Reshape3/1
  Hrw/1 -> Reshape10/1
  Reshape10/1 -> IC3/1
  Reshape2/1 -> IC4/1
  wRW/1 -> Reshape2/1
  Reshape3/1 -> w_RW_B/1
  Reshape11/1 -> Product3/2
  Hrw_dot_1/1 -> Reshape11/1
  Product3/1 -> Reshape1/1

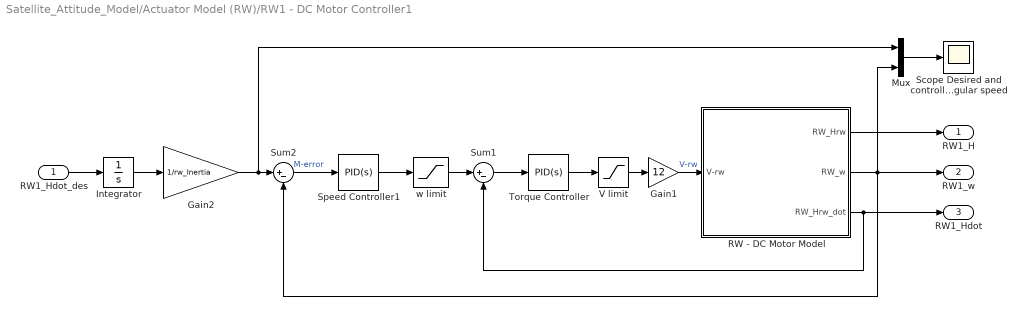
== system Satellite_Attitude_Model/Actuator Model (RW)/RW1 - DC Motor Controller1 ==
  RW1_Hdot_des : Inport
  Gain1 : Gain  Gain=12
  Gain2 : Gain  Gain=1/rw_Inertia
  Integrator : Integrator
  Mux : Mux  Inputs=2
  RW - DC Motor Model : Subsystem
  "Scope Desired and controlled RW-angular speed " : Scope
  Speed Controller1 : simulink/Continuous/PID Controller  Controller=PID  Form=Parallel  TimeDomain=Continuous-time  SampleTime=0.01  IntegratorMethod=Forward Euler  FilterMethod=Forward Euler  ControllerParametersSource=internal  P=9.56052273582853  I=13.4366327144231  D=1.16248121318414  UseFilter=on  N=2668.95305381072  TunerSelectOption=Transfer Function Based (PID Tuner App)  InitialConditionSource=internal  InitialConditionForIntegrator=0  InitialConditionForFilter=0  DifferentiatorICPrevScaledInput=0  ExternalReset=none  TrackingMode=off  Kt=1  LimitOutput=off  UpperSaturationLimit=inf  LowerSaturationLimit=-inf  LinearizeAsGain=on  AntiWindupMode=none  Kb=1  POutMin=[]  POutMax=[]  IOutMin=[]  IOutMax=[]  DOutMin=[]  DOutMax=[]  NOutMin=[]  NOutMax=[]  SumOutMin=[]  SumOutMax=[]  SaturationOutMin=[]  SaturationOutMax=[]  PParamMin=[]  PParamMax=[]  IParamMin=[]  IParamMax=[]  DParamMin=[]  DParamMax=[]  NParamMin=[]  NParamMax=[]  KbParamMin=[]  KbParamMax=[]  KtParamMin=[]  KtParamMax=[]  KbOutMin=[]  KbOutMax=[]  KtOutMin=[]  KtOutMax=[]  IntegratorOutMin=[]  IntegratorOutMax=[]  FilterOutMin=[]  FilterOutMax=[]  SumI1OutMin=[]  SumI1OutMax=[]  SumI2OutMin=[]  SumI2OutMax=[]  SumI3OutMin=[]  SumI3OutMax=[]  SumI4OutMin=[]  SumI4OutMax=[]  SumDOutMin=[]  SumDOutMax=[]  DifferentiatorOutMin=[]  DifferentiatorOutMax=[]  FilterDiffOutCoefMin=[]  FilterDiffOutCoefMax=[]  ReciprocalOutMin=[]  ReciprocalOutMax=[]  SumDenOutMin=[]  SumDenOutMax=[]  SumNumOutMin=[]  SumNumOutMax=[]  DivideOutMin=[]  DivideOutMax=[]  IntegratorContinuousStateAttributes=''  IntegratorStateMustResolveToSignalObject=off  IntegratorRTWStateStorageClass=Auto  FilterContinuousStateAttributes=''  FilterStateMustResolveToSignalObject=off  FilterRTWStateStorageClass=Auto  ParallelPVariant=InternalParameters  IdealPVariant=Disabled  IVariant=InternalParameters  DVariant=InternalParameters  IntegratorVariant=Continuous  SatVariant=Disabled  AWVariant=Passthrough  PCopyVariant=Disabled  TRVariant=Disabled  FdbkBlocksVariant=Forward  IdealPFdbkVariant=Disabled  SatFdbkVariant=Disabled  DerivativeFilterVariant=ContFilter  NVariant=InternalParameters  NCopyVariant=Disabled  FilterICVariant=InternalICsFilter  IntegratorICVariant=InternalICs  ExternalResetVariant=Disabled  TRSumVariant=Passthrough  SumFdbkVariant=Disabled  SumVariant=Sum_PID
  Sum1 : Sum  Inputs=|+-
  Sum2 : Sum  Inputs=|+-
  Torque Controller : simulink/Continuous/PID Controller  Controller=PID  Form=Parallel  TimeDomain=Continuous-time  SampleTime=0.01  IntegratorMethod=Forward Euler  FilterMethod=Forward Euler  ControllerParametersSource=internal  P=2.50374683332827e-05  I=0.022215359014968  D=0  UseFilter=on  N=100  TunerSelectOption=Transfer Function Based (PID Tuner App)  InitialConditionSource=internal  InitialConditionForIntegrator=0  InitialConditionForFilter=0  DifferentiatorICPrevScaledInput=0  ExternalReset=none  TrackingMode=off  Kt=1  LimitOutput=off  UpperSaturationLimit=inf  LowerSaturationLimit=-inf  LinearizeAsGain=on  AntiWindupMode=none  Kb=1  POutMin=[]  POutMax=[]  IOutMin=[]  IOutMax=[]  DOutMin=[]  DOutMax=[]  NOutMin=[]  NOutMax=[]  SumOutMin=[]  SumOutMax=[]  SaturationOutMin=[]  SaturationOutMax=[]  PParamMin=[]  PParamMax=[]  IParamMin=[]  IParamMax=[]  DParamMin=[]  DParamMax=[]  NParamMin=[]  NParamMax=[]  KbParamMin=[]  KbParamMax=[]  KtParamMin=[]  KtParamMax=[]  KbOutMin=[]  KbOutMax=[]  KtOutMin=[]  KtOutMax=[]  IntegratorOutMin=[]  IntegratorOutMax=[]  FilterOutMin=[]  FilterOutMax=[]  SumI1OutMin=[]  SumI1OutMax=[]  SumI2OutMin=[]  SumI2OutMax=[]  SumI3OutMin=[]  SumI3OutMax=[]  SumI4OutMin=[]  SumI4OutMax=[]  SumDOutMin=[]  SumDOutMax=[]  DifferentiatorOutMin=[]  DifferentiatorOutMax=[]  FilterDiffOutCoefMin=[]  FilterDiffOutCoefMax=[]  ReciprocalOutMin=[]  ReciprocalOutMax=[]  SumDenOutMin=[]  SumDenOutMax=[]  SumNumOutMin=[]  SumNumOutMax=[]  DivideOutMin=[]  DivideOutMax=[]  IntegratorContinuousStateAttributes=''  IntegratorStateMustResolveToSignalObject=off  IntegratorRTWStateStorageClass=Auto  FilterContinuousStateAttributes=''  FilterStateMustResolveToSignalObject=off  FilterRTWStateStorageClass=Auto  ParallelPVariant=InternalParameters  IdealPVariant=Disabled  IVariant=InternalParameters  DVariant=InternalParameters  IntegratorVariant=Continuous  SatVariant=Disabled  AWVariant=Passthrough  PCopyVariant=Disabled  TRVariant=Disabled  FdbkBlocksVariant=Forward  IdealPFdbkVariant=Disabled  SatFdbkVariant=Disabled  DerivativeFilterVariant=ContFilter  NVariant=InternalParameters  NCopyVariant=Disabled  FilterICVariant=InternalICsFilter  IntegratorICVariant=InternalICs  ExternalResetVariant=Disabled  TRSumVariant=Passthrough  SumFdbkVariant=Disabled  SumVariant=Sum_PID
  V limit : Saturate  UpperLimit=20  LowerLimit=-20
  w limit : Saturate  UpperLimit=RW_wmax  LowerLimit=-RW_wmax
  RW1_H : Outport
  RW1_w : Outport  Port=2
  RW1_Hdot : Outport  Port=3
  wires:
  Torque Controller/1 -> V limit/1
  RW - DC Motor Model/3(RW_Hrw_dot) -> RW1_Hdot/1, Sum1/2
  Mux/1 -> "Scope Desired and controlled RW-angular speed "/1
  V limit/1 -> Gain1/1
  Gain1/1 -> RW - DC Motor Model/1(V-rw)  "V-rw"
  RW - DC Motor Model/2(RW_w) -> RW1_w/1, Sum2/2, Mux/2
  Sum1/1 -> Torque Controller/1
  RW - DC Motor Model/1(RW_Hrw) -> RW1_H/1
  Speed Controller1/1 -> w limit/1
  w limit/1 -> Sum1/1
  Sum2/1 -> Speed Controller1/1  "M-error"
  Integrator/1 -> Gain2/1
  RW1_Hdot_des/1 -> Integrator/1
  Gain2/1 -> Mux/1, Sum2/1

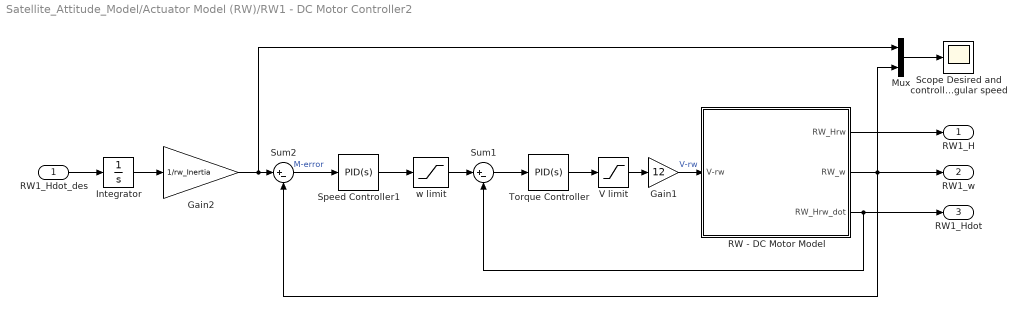
== system Satellite_Attitude_Model/Actuator Model (RW)/RW1 - DC Motor Controller2 ==
  RW1_Hdot_des : Inport
  Gain1 : Gain  Gain=12
  Gain2 : Gain  Gain=1/rw_Inertia
  Integrator : Integrator
  Mux : Mux  Inputs=2
  RW - DC Motor Model : Subsystem
  "Scope Desired and controlled RW-angular speed " : Scope
  Speed Controller1 : simulink/Continuous/PID Controller  Controller=PID  Form=Parallel  TimeDomain=Continuous-time  SampleTime=0.01  IntegratorMethod=Forward Euler  FilterMethod=Forward Euler  ControllerParametersSource=internal  P=9.56052273582853  I=13.4366327144231  D=1.16248121318414  UseFilter=on  N=2668.95305381072  TunerSelectOption=Transfer Function Based (PID Tuner App)  InitialConditionSource=internal  InitialConditionForIntegrator=0  InitialConditionForFilter=0  DifferentiatorICPrevScaledInput=0  ExternalReset=none  TrackingMode=off  Kt=1  LimitOutput=off  UpperSaturationLimit=inf  LowerSaturationLimit=-inf  LinearizeAsGain=on  AntiWindupMode=none  Kb=1  POutMin=[]  POutMax=[]  IOutMin=[]  IOutMax=[]  DOutMin=[]  DOutMax=[]  NOutMin=[]  NOutMax=[]  SumOutMin=[]  SumOutMax=[]  SaturationOutMin=[]  SaturationOutMax=[]  PParamMin=[]  PParamMax=[]  IParamMin=[]  IParamMax=[]  DParamMin=[]  DParamMax=[]  NParamMin=[]  NParamMax=[]  KbParamMin=[]  KbParamMax=[]  KtParamMin=[]  KtParamMax=[]  KbOutMin=[]  KbOutMax=[]  KtOutMin=[]  KtOutMax=[]  IntegratorOutMin=[]  IntegratorOutMax=[]  FilterOutMin=[]  FilterOutMax=[]  SumI1OutMin=[]  SumI1OutMax=[]  SumI2OutMin=[]  SumI2OutMax=[]  SumI3OutMin=[]  SumI3OutMax=[]  SumI4OutMin=[]  SumI4OutMax=[]  SumDOutMin=[]  SumDOutMax=[]  DifferentiatorOutMin=[]  DifferentiatorOutMax=[]  FilterDiffOutCoefMin=[]  FilterDiffOutCoefMax=[]  ReciprocalOutMin=[]  ReciprocalOutMax=[]  SumDenOutMin=[]  SumDenOutMax=[]  SumNumOutMin=[]  SumNumOutMax=[]  DivideOutMin=[]  DivideOutMax=[]  IntegratorContinuousStateAttributes=''  IntegratorStateMustResolveToSignalObject=off  IntegratorRTWStateStorageClass=Auto  FilterContinuousStateAttributes=''  FilterStateMustResolveToSignalObject=off  FilterRTWStateStorageClass=Auto  ParallelPVariant=InternalParameters  IdealPVariant=Disabled  IVariant=InternalParameters  DVariant=InternalParameters  IntegratorVariant=Continuous  SatVariant=Disabled  AWVariant=Passthrough  PCopyVariant=Disabled  TRVariant=Disabled  FdbkBlocksVariant=Forward  IdealPFdbkVariant=Disabled  SatFdbkVariant=Disabled  DerivativeFilterVariant=ContFilter  NVariant=InternalParameters  NCopyVariant=Disabled  FilterICVariant=InternalICsFilter  IntegratorICVariant=InternalICs  ExternalResetVariant=Disabled  TRSumVariant=Passthrough  SumFdbkVariant=Disabled  SumVariant=Sum_PID
  Sum1 : Sum  Inputs=|+-
  Sum2 : Sum  Inputs=|+-
  Torque Controller : simulink/Continuous/PID Controller  Controller=PID  Form=Parallel  TimeDomain=Continuous-time  SampleTime=0.01  IntegratorMethod=Forward Euler  FilterMethod=Forward Euler  ControllerParametersSource=internal  P=2.50374683332827e-05  I=0.022215359014968  D=0  UseFilter=on  N=100  TunerSelectOption=Transfer Function Based (PID Tuner App)  InitialConditionSource=internal  InitialConditionForIntegrator=0  InitialConditionForFilter=0  DifferentiatorICPrevScaledInput=0  ExternalReset=none  TrackingMode=off  Kt=1  LimitOutput=off  UpperSaturationLimit=inf  LowerSaturationLimit=-inf  LinearizeAsGain=on  AntiWindupMode=none  Kb=1  POutMin=[]  POutMax=[]  IOutMin=[]  IOutMax=[]  DOutMin=[]  DOutMax=[]  NOutMin=[]  NOutMax=[]  SumOutMin=[]  SumOutMax=[]  SaturationOutMin=[]  SaturationOutMax=[]  PParamMin=[]  PParamMax=[]  IParamMin=[]  IParamMax=[]  DParamMin=[]  DParamMax=[]  NParamMin=[]  NParamMax=[]  KbParamMin=[]  KbParamMax=[]  KtParamMin=[]  KtParamMax=[]  KbOutMin=[]  KbOutMax=[]  KtOutMin=[]  KtOutMax=[]  IntegratorOutMin=[]  IntegratorOutMax=[]  FilterOutMin=[]  FilterOutMax=[]  SumI1OutMin=[]  SumI1OutMax=[]  SumI2OutMin=[]  SumI2OutMax=[]  SumI3OutMin=[]  SumI3OutMax=[]  SumI4OutMin=[]  SumI4OutMax=[]  SumDOutMin=[]  SumDOutMax=[]  DifferentiatorOutMin=[]  DifferentiatorOutMax=[]  FilterDiffOutCoefMin=[]  FilterDiffOutCoefMax=[]  ReciprocalOutMin=[]  ReciprocalOutMax=[]  SumDenOutMin=[]  SumDenOutMax=[]  SumNumOutMin=[]  SumNumOutMax=[]  DivideOutMin=[]  DivideOutMax=[]  IntegratorContinuousStateAttributes=''  IntegratorStateMustResolveToSignalObject=off  IntegratorRTWStateStorageClass=Auto  FilterContinuousStateAttributes=''  FilterStateMustResolveToSignalObject=off  FilterRTWStateStorageClass=Auto  ParallelPVariant=InternalParameters  IdealPVariant=Disabled  IVariant=InternalParameters  DVariant=InternalParameters  IntegratorVariant=Continuous  SatVariant=Disabled  AWVariant=Passthrough  PCopyVariant=Disabled  TRVariant=Disabled  FdbkBlocksVariant=Forward  IdealPFdbkVariant=Disabled  SatFdbkVariant=Disabled  DerivativeFilterVariant=ContFilter  NVariant=InternalParameters  NCopyVariant=Disabled  FilterICVariant=InternalICsFilter  IntegratorICVariant=InternalICs  ExternalResetVariant=Disabled  TRSumVariant=Passthrough  SumFdbkVariant=Disabled  SumVariant=Sum_PID
  V limit : Saturate  UpperLimit=20  LowerLimit=-20
  w limit : Saturate  UpperLimit=RW_wmax  LowerLimit=-RW_wmax
  RW1_H : Outport
  RW1_w : Outport  Port=2
  RW1_Hdot : Outport  Port=3
  wires:
  Torque Controller/1 -> V limit/1
  RW - DC Motor Model/3(RW_Hrw_dot) -> RW1_Hdot/1, Sum1/2
  Mux/1 -> "Scope Desired and controlled RW-angular speed "/1
  V limit/1 -> Gain1/1
  Gain1/1 -> RW - DC Motor Model/1(V-rw)  "V-rw"
  RW - DC Motor Model/2(RW_w) -> RW1_w/1, Sum2/2, Mux/2
  Sum1/1 -> Torque Controller/1
  RW - DC Motor Model/1(RW_Hrw) -> RW1_H/1
  Speed Controller1/1 -> w limit/1
  w limit/1 -> Sum1/1
  Sum2/1 -> Speed Controller1/1  "M-error"
  Integrator/1 -> Gain2/1
  RW1_Hdot_des/1 -> Integrator/1
  Gain2/1 -> Mux/1, Sum2/1
